simulink model "sim_dinamica"  (R2020a)
settings: Solver=VariableStepAuto  StartTime=0.0  StopTime=25  RelTol=1e-3
undefined symbols (not defined in the file): theta_initial, torque_final, torque_initial, torque_step_time
(part 3 of 3)

== matlab function sim_dinamica/MATLAB Function ==
  data: dTh input; F output
function F = calcul_F(dTh)

F = 1.2*dTh;
